simulink model "SAR_output"  (R2018b)
settings: Solver=VariableStepAuto  StartTime=0.0  StopTime=10.0  RelTol=1e-3
settings Model: Creator=iamcy  LastModifiedBy=iamcy

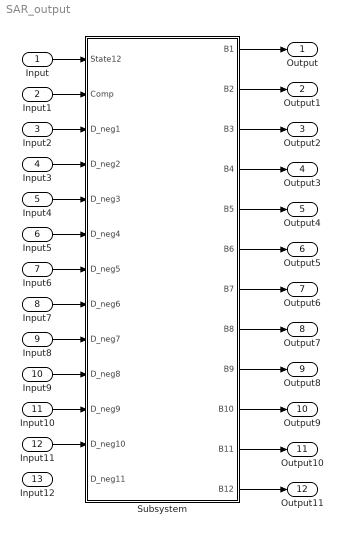
== system SAR_output ==
  Input : Inport
  Input1 : Inport  Port=2
  Input2 : Inport  Port=3
  Input3 : Inport  Port=4
  Input4 : Inport  Port=5
  Input5 : Inport  Port=6
  Input6 : Inport  Port=7
  Input7 : Inport  Port=8
  Input8 : Inport  Port=9
  Input9 : Inport  Port=10
  Input10 : Inport  Port=11
  Input11 : Inport  Port=12
  Input12 : Inport  Port=13
  Subsystem : Subsystem
  Output : Outport
  Output1 : Outport  Port=2
  Output2 : Outport  Port=3
  Output3 : Outport  Port=4
  Output4 : Outport  Port=5
  Output5 : Outport  Port=6
  Output6 : Outport  Port=7
  Output7 : Outport  Port=8
  Output8 : Outport  Port=9
  Output9 : Outport  Port=10
  Output10 : Outport  Port=11
  Output11 : Outport  Port=12
  wires:
  Subsystem/1(B1) -> Output/1
  Subsystem/2(B2) -> Output1/1
  Subsystem/3(B3) -> Output2/1
  Subsystem/4(B4) -> Output3/1
  Subsystem/6(B6) -> Output5/1
  Subsystem/5(B5) -> Output4/1
  Subsystem/7(B7) -> Output6/1
  Subsystem/8(B8) -> Output7/1
  Subsystem/9(B9) -> Output8/1
  Subsystem/10(B10) -> Output9/1
  Subsystem/11(B11) -> Output10/1
  Subsystem/12(B12) -> Output11/1
  Input/1 -> Subsystem/1(State12)
  Input1/1 -> Subsystem/2(Comp)
  Input2/1 -> Subsystem/3(D_neg1)
  Input3/1 -> Subsystem/4(D_neg2)
  Input4/1 -> Subsystem/5(D_neg3)
  Input5/1 -> Subsystem/6(D_neg4)
  Input6/1 -> Subsystem/7(D_neg5)
  Input7/1 -> Subsystem/8(D_neg6)
  Input8/1 -> Subsystem/9(D_neg7)
  Input9/1 -> Subsystem/10(D_neg8)
  Input10/1 -> Subsystem/11(D_neg9)
  Input11/1 -> Subsystem/12(D_neg10)

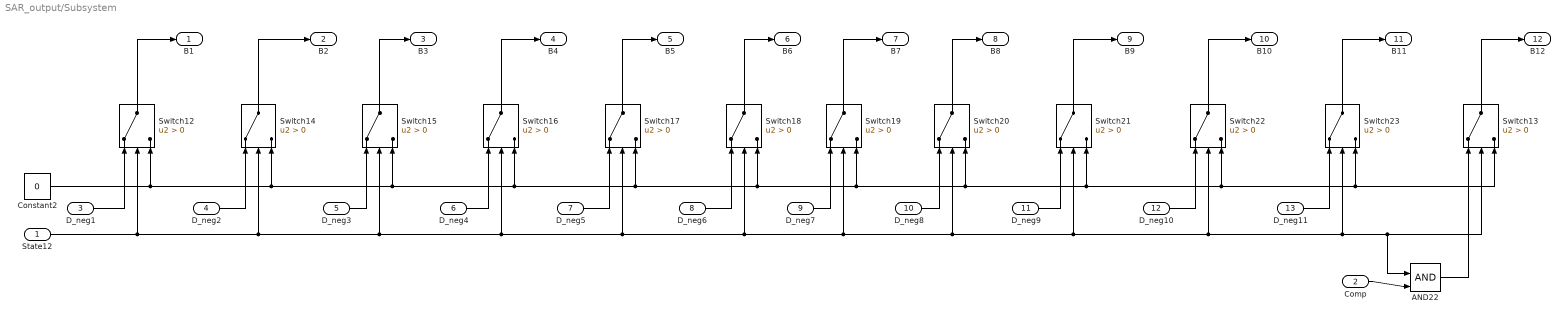
== system SAR_output/Subsystem ==
  State12 : Inport
  Comp : Inport  Port=2
  D_neg1 : Inport  Port=3
  D_neg2 : Inport  Port=4
  D_neg3 : Inport  Port=5
  D_neg4 : Inport  Port=6
  D_neg5 : Inport  Port=7
  D_neg6 : Inport  Port=8
  D_neg7 : Inport  Port=9
  D_neg8 : Inport  Port=10
  D_neg9 : Inport  Port=11
  D_neg10 : Inport  Port=12
  D_neg11 : Inport  Port=13
  AND22 : Logic  IconShape=distinctive  AllPortsSameDT=off  OutDataTypeStr=boolean
  Constant2 : Constant  Value=0
  Switch{12..23} (12 alike) : Switch  Criteria=u2 > Threshold
  B1 : Outport
  B2 : Outport  Port=2
  B3 : Outport  Port=3
  B4 : Outport  Port=4
  B5 : Outport  Port=5
  B6 : Outport  Port=6
  B7 : Outport  Port=7
  B8 : Outport  Port=8
  B9 : Outport  Port=9
  B10 : Outport  Port=10
  B11 : Outport  Port=11
  B12 : Outport  Port=12
  wires:
  Constant2/1 -> Switch12/3, Switch13/3, Switch23/3, Switch22/3, Switch21/3, Switch20/3, Switch19/3, Switch18/3, Switch17/3, Switch16/3, Switch15/3, Switch14/3
  Switch22/1 -> B10/1
  Switch17/1 -> B5/1
  Switch12/1 -> B1/1
  Switch14/1 -> B2/1
  Switch18/1 -> B6/1
  Switch16/1 -> B4/1
  Switch15/1 -> B3/1
  Switch23/1 -> B11/1
  Switch20/1 -> B8/1
  Switch21/1 -> B9/1
  Switch19/1 -> B7/1
  Switch13/1 -> B12/1
  State12/1 -> Switch12/2, Switch14/2, Switch15/2, Switch16/2, Switch17/2, Switch19/2, Switch20/2, Switch21/2, Switch22/2, AND22/1, Switch13/2, Switch23/2, Switch18/2
  AND22/1 -> Switch13/1
  Comp/1 -> AND22/2
  D_neg11/1 -> Switch23/1
  D_neg10/1 -> Switch22/1
  D_neg9/1 -> Switch21/1
  D_neg8/1 -> Switch20/1
  D_neg7/1 -> Switch19/1
  D_neg6/1 -> Switch18/1
  D_neg5/1 -> Switch17/1
  D_neg4/1 -> Switch16/1
  D_neg3/1 -> Switch15/1
  D_neg2/1 -> Switch14/1
  D_neg1/1 -> Switch12/1
